simulink model "quadcopter_swarm_final_solution"  (R2023b)
settings: Solver=ode3  StartTime=0  StopTime=inf  FixedStep=0.005  RelTol=1e-3  EnableMultiTasking=on
values from neighbouring files (symbols this model uses):
  angle_outer_max = 60    [1nrx_dot.mat]    (also in 1nrxdrones_dot.mat; collision_avoidance_POS.mat; collision_avoidance_headonfix_POS.mat; collision_test.mat)
  F_e_g = [0 0 39.28]    [1nrx_dot.mat]    (also in 1nrxdrones_dot.mat; collision_avoidance_POS.mat; collision_avoidance_headonfix_POS.mat; collision_test.mat)
  g = 9.82    [1nrx_dot.mat]    (also in 1nrxdrones_dot.mat; collision_avoidance_POS.mat; collision_avoidance_headonfix_POS.mat; collision_test.mat)
  I_C = [0.5  0  0; 0  0.5  0; 0  0  1]    [1nrx_dot.mat]    (also in 1nrxdrones_dot.mat; collision_avoidance_POS.mat; collision_avoidance_headonfix_POS.mat; collision_test.mat)
  in_D = 20    [1nrx_dot.mat]    (also in 1nrxdrones_dot.mat; collision_avoidance_POS.mat; collision_avoidance_headonfix_POS.mat; collision_test.mat)
  in_I = 0    [1nrx_dot.mat]    (also in 1nrxdrones_dot.mat; collision_avoidance_POS.mat; collision_avoidance_headonfix_POS.mat; collision_test.mat)
  in_P = 20    [1nrx_dot.mat]    (also in 1nrxdrones_dot.mat; collision_avoidance_POS.mat; collision_avoidance_headonfix_POS.mat; collision_test.mat)
  in_thrust_D = 30    [1nrx_dot.mat]    (also in 1nrxdrones_dot.mat; collision_avoidance_POS.mat; collision_avoidance_headonfix_POS.mat; collision_test.mat)
  in_thrust_I = 0    [1nrx_dot.mat]    (also in 1nrxdrones_dot.mat; collision_avoidance_POS.mat; collision_avoidance_headonfix_POS.mat; collision_test.mat)
  in_thrust_P = 10    [1nrx_dot.mat]    (also in 1nrxdrones_dot.mat; collision_avoidance_POS.mat; collision_avoidance_headonfix_POS.mat; collision_test.mat)
  L = [4 -1 -1 -1 -1 0 -1 4 -1 -1 -1 0 ... (36 elements, 6x6)]    [1nrx_dot.mat]    (also in 1nrxdrones_dot.mat; collision_avoidance_POS.mat; collision_avoidance_headonfix_POS.mat; collision_test.mat)
  m = 4    [1nrx_dot.mat]    (also in 1nrxdrones_dot.mat; collision_avoidance_POS.mat; collision_avoidance_headonfix_POS.mat; collision_test.mat)
  M_RB = [4 0 0 0 0 0 0 4 0 0 0 0 ... (36 elements, 6x6)]    [1nrx_dot.mat]    (also in 1nrxdrones_dot.mat; collision_avoidance_POS.mat; collision_avoidance_headonfix_POS.mat; collision_test.mat)
  p_0 = [5  10; 5  -5; -8  5; 5  -13; 8  8; 0  0]    [1nrx_dot.mat]    (also in 1nrxdrones_dot.mat; collision_avoidance_POS.mat; collision_avoidance_headonfix_POS.mat; collision_test.mat)
  p_d = [1  0; 4  0; -2  0; 7  0; 9  0; 0  0]    [1nrx_dot.mat]    (also in 1nrxdrones_dot.mat; collision_avoidance_POS.mat; collision_avoidance_headonfix_POS.mat; collision_test.mat)
  R_c = 3    [1nrx_dot.mat]    (also in 1nrxdrones_dot.mat; collision_avoidance_POS.mat; collision_avoidance_headonfix_POS.mat; collision_test.mat)
  r_m = 2.2    [1nrx_dot.mat]    (also in 1nrxdrones_dot.mat; collision_avoidance_POS.mat; collision_avoidance_headonfix_POS.mat; collision_test.mat)
  thrust_max = 196.4    [1nrx_dot.mat]    (also in 1nrxdrones_dot.mat; collision_avoidance_POS.mat; collision_avoidance_headonfix_POS.mat; collision_test.mat)
  V = [1 2 3 4 5 6]    [1nrx_dot.mat]    (also in 1nrxdrones_dot.mat; collision_avoidance_POS.mat; collision_avoidance_headonfix_POS.mat; collision_test.mat)
  v_angle_in_max = 60    [1nrx_dot.mat]    (also in 1nrxdrones_dot.mat; collision_avoidance_POS.mat; collision_avoidance_headonfix_POS.mat; collision_test.mat)
  w = 0.6    [1nrx_dot.mat]    (also in 1nrxdrones_dot.mat; collision_avoidance_POS.mat; collision_avoidance_headonfix_POS.mat; collision_test.mat)
  w_1 = 6    [1nrx_dot.mat]    (also in 1nrxdrones_dot.mat; collision_avoidance_POS.mat; collision_avoidance_headonfix_POS.mat; collision_test.mat)
  w_2_with_h = 2.56430849099    [1nrx_dot.mat]    (also in 1nrxdrones_dot.mat; collision_avoidance_POS.mat; collision_avoidance_headonfix_POS.mat; collision_test.mat)
libraries: simulink_extras x37, slpidlib x30, sharedtransform x27, aerolibutil x25, dspsigops x24, dspindex x13, sharedutil x5, vrlib x2
(part 1 of 7)
settings Model: Creator=The MathWorks, Inc.  LastModifiedBy=Søren
settings SolverCC: AlgebraicLoopSolver=TrustRegion
settings DataIOCC: LimitDataPoints=on  SaveFormat=Array  SaveOutput=off  SignalLogging=off  DSMLogging=off  SaveTime=off  ReturnWorkspaceOutputs=off
settings OptimizationCC: BlockReduction=off  BufferReuse=off  LifeSpan=inf
settings DebuggingCC: AlgebraicLoopMsg=none  ParameterPrecisionLossMsg=none  AllowSymbolicDim=off  PregeneratedLibrarySubsystemCodeDiagnostic=none  SFUnexpectedBacktrackingDiag=warning  SFNoUnconditionalDefaultTransitionDiag=warning  SFExecutionAtInitializationDiag=none  ArithmeticOperatorsInVariantConditions=warning
settings HardwareCC: ProdBitPerPointer=32  ProdBitPerSizeT=32  ProdBitPerPtrDiffT=32  ProdLargestAtomicFloat=None  ProdIntDivRoundTo=Undefined  ProdEndianess=Unspecified  ProdWordSize=32  ProdHWDeviceType=32-bit Generic
settings ModelReferenceCC: EnableRefExpFcnMdlSchedulingChecks=on  PropagateSignalLabelsOutOfModel=off
settings SFSimCC: SimUseLocalCustomCode=off  CustomCodeUndefinedFunction=UseInterfaceOnly
settings RTWCC: RTWUseLocalCustomCode=off  DLArmComputeVersion=19.05
settings CodeAppCC: StateflowObjectComments=on
settings GRTTargetCC: TargetLangStandard=C89/C90 (ANSI)
settings ConfigComp: CovMetricSettings=dw  CovSaveCumulativeToWorkspaceVar=on  CovSaveSingleToWorkspaceVar=on  CovExternalEMLEnable=off  CovSFcnEnable=off

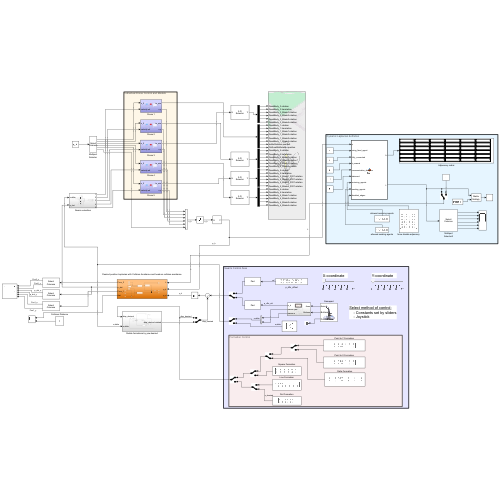
[thumbnail: Simulink's stored preview of the top-level diagram]
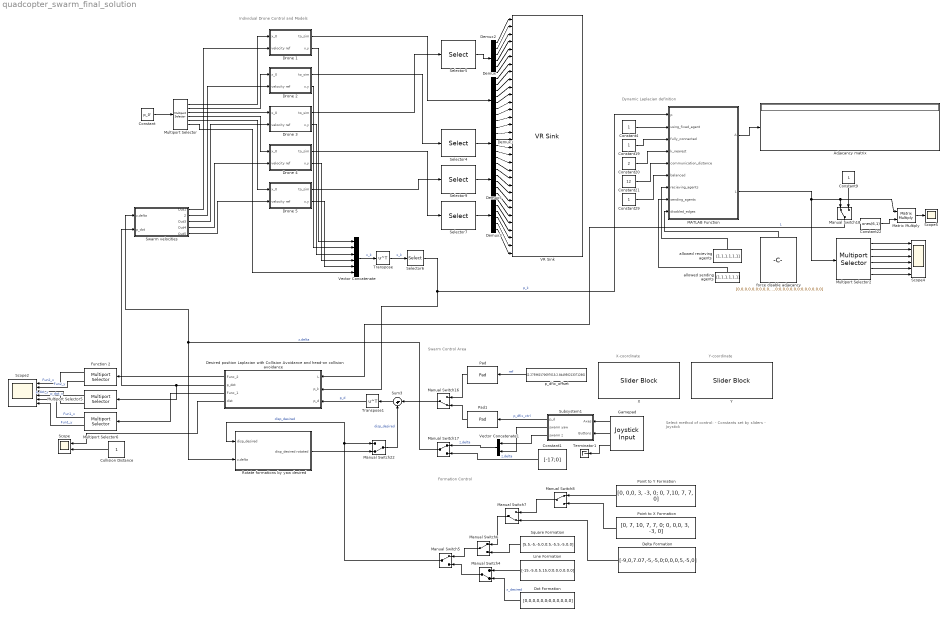
== system quadcopter_swarm_final_solution ==
  note: Individual Drone Control and Models
  note: Select method of control:
      | - Constants set by sliders
      | - Joystick
  note: Formation Control
  note: Swarm Control Area
  note: Dynamic Laplacian definition
  note: X-coordinate
  note: Y-coordinate
  Adjacancy matrix : Display
  Collision Distance : Constant
  Constant : Constant  Value=p_0'
  Constant1 : Constant  Value=[-17;0]  VectorParams1D=off
  Constant19 : Constant
  Constant20 : Constant  Value=2
  Constant21 : Constant  Value=12
  Constant22 : Constant  Value=ones(6,1)
  Constant29 : Constant
  Constant4 : Constant
  Constant9 : Constant  Value=L
  Delta Formation : Constant  Value=[-9,0,7.07,-5,-5,0;0,0,0,5,-5,0]
  Demux : Demux  Outputs=8
  Demux{1..3,5} (4 alike) : Demux  Outputs=6
  "Desired position Laplacian with Collision Avoidance and head-on collision avoidance " : Subsystem
  Dot Formation : Constant  Value=[0,0,0,0,0,0;0,0,0,0,0,0]
  Drone 1 : Subsystem
  Drone 2 : Subsystem
  Drone 3 : Subsystem
  Drone 4 : Subsystem
  Drone 5 : Subsystem
  Function 2 : dspindex/Multiport Selector  rowsOrCols=Columns  idxCellArray={ 1,2 }  idxErrMode=Clip Index
      settings: LibrarySourceBlock=|
      | dsphdlsupportsigmgmt/Multiport
      | Selector
  Gamepad : vrlib/Joystick Input  joyid=1  adjustports=on  forcefeed=off
  Line Formation : Constant  Value=[-15,-5,0,5,15,0;0,0,0,0,0,0]
  MATLAB Function : MATLAB Function  TreatAsAtomicUnit=on
  Manual Switch{4,7,16,22} (4 alike) : ManualSwitch  CurrentSetting=0
  Manual Switch{5..6,8,17..18} (5 alike) : ManualSwitch
  Matrix Multiply : Product  Multiplication=Matrix(*)
  Multiport Selector : dspindex/Multiport Selector  rowsOrCols=Columns  idxCellArray={1,2,3,4,5,6}  idxErrMode=Clip Index
      settings: LibrarySourceBlock=|
      | dsphdlsupportsigmgmt/Multiport
      | Selector
  Multiport Selector2 : dspindex/Multiport Selector  rowsOrCols=Columns  idxCellArray={ 1,2,3,4,5,6}  idxErrMode=Clip Index
      settings: LibrarySourceBlock=|
      | dsphdlsupportsigmgmt/Multiport
      | Selector
  Multiport Selector5 : dspindex/Multiport Selector  rowsOrCols=Columns  idxCellArray={ 1,2 }  idxErrMode=Clip Index
      settings: LibrarySourceBlock=|
      | dsphdlsupportsigmgmt/Multiport
      | Selector
  Multiport Selector6 : dspindex/Multiport Selector  rowsOrCols=Columns  idxCellArray={ 1,2 }  idxErrMode=Clip Index
      settings: LibrarySourceBlock=|
      | dsphdlsupportsigmgmt/Multiport
      | Selector
  Pad : dspsigops/Pad  padAlong=Rows  dimsToPad=1  valSrc=Specify via dialog  padVal=0  spec=Output size  padNumOutRowsSpecMethod=User-specified  numOutRows=2  padNumOutColsSpecMethod=User-specified  numOutCols=size(p_d,1)  isVarDimsMode=off  padBeginning=0  padEnd=0  outSizeMode=User-specified  outSize=1  padSigAt=Beginning  trunc_flag=None  roundingMode=Floor  overflowMode=off  truncOrWrapMode=Truncate  wrap_flag=None
  Pad1 : dspsigops/Pad  padAlong=Rows  dimsToPad=1  valSrc=Specify via dialog  padVal=0  spec=Output size  padNumOutRowsSpecMethod=User-specified  numOutRows=2  padNumOutColsSpecMethod=User-specified  numOutCols=size(p_d,1)  isVarDimsMode=off  padBeginning=0  padEnd=0  outSizeMode=User-specified  outSize=1  padSigAt=Beginning  trunc_flag=None  roundingMode=Floor  overflowMode=off  truncOrWrapMode=Truncate  wrap_flag=None
  Point to X Formation : Constant  Value=[0, 7, 10, 7, 7, 0; 0, 0,0, 3, -3, 0]
  Point to Y Formation : Constant  Value=[0, 0,0, 3, -3, 0; 0, 7,10, 7, 7, 0]
  Rotate formations by yaw desired : Subsystem
  Scope : Scope  NumInputPorts=2
  Scope2 : Scope  NumInputPorts=6
  Scope4 : Scope  NumInputPorts=6
  Scope5 : Scope
  Selector{4..5,7,9} (4 alike) : Selector  NumberOfDimensions=2  InputPortWidth=8  IndexOptions=Index vector (dialog),Select all  Indices=1:23,1  OutputSizes=1,1
  Selector6 : Selector  NumberOfDimensions=2  InputPortWidth=3  IndexOptions=Index vector (dialog),Select all  Indices=V,1  OutputSizes=1,1
  Square Formation : Constant  Value=[5,5,-5,-5,0,0;5,-5,5,-5,0,0]  VectorParams1D=off
  Subsystem1 : Subsystem
  Sum3 : Sum  Inputs=|-+
  Swarm velocities : Subsystem
  Terminator1 : Terminator
  Transpose : Math  Operator=transpose
  Transpose1 : Math  Operator=transpose
  VR Sink : vrlib/VR Sink  InstantiateOnLoad=on  SampleTime=12*0.005  ViewEnable=on  RemoteChange=off  RemoteView=off  FieldsWritten=QuadBody_3.rotation.4.1.1.double#QuadBody_3.translation.3.1.1.double#QuadBody_3_Blade1.rotation.4.1.1.double#QuadBody_3_Blade3.rotation.4.1.1.double#QuadBody_3_Blade2.rotation.4.1.1.double#QuadBody_3_Blade4.rotation.4.1.1.double#QuadBody_1.rotation.4.1.1.double#QuadBody_1.translation.3.1.1.double#QuadBody_1_Blade1.rotation.4.1.1.double#QuadBody_1_Blade3.rotation.4.1.1.double#QuadBody_1_Blade2.rotation.4.1.1.double#QuadBody_1_Blade4.rotation.4.1.1.double#IsoNoRotation.position.3.1.1.double#OnQuadNoRotation.position.3.1.1.double#QuadBody_2.rotation.4.1.1.double#QuadBody_2.translation.3.1.1.double#QuadBody_2_Blade1.rotation.4.1.1.double#QuadBody_2_Blade3.rotation.4.1.1.double#QuadBody_2_Blade2.rotation.4.1.1.double#QuadBody_2_Blade4.rotation.4.1.1.double#QuadBody_5.rotation.4.1.1.double#QuadBody_5.translation.3.1.1.double#QuadBody_5_Blade1_0001.rotation.4.1.1.double#QuadBody_5_Blade3_0001.rotation.4.1.1.double#QuadBody_5_Blade2_0001.rotation.4.1.1.double#QuadBody_5_Blade4_0001.rotation.4.1.1.double#QuadBody_4.rotation.4.1.1.double#QuadBody_4.translation.3.1.1.double#QuadBody_4_Blade1.rotation.4.1.1.double#QuadBody_4_Blade3.rotation.4.1.1.double#QuadBody_4_Blade2.rotation.4.1.1.double#QuadBody_4_Blade4.rotation.4.1.1.double  WorldFileName=Quadcopter_VR.wrl  AutoView=on  VideoDimensions=[]  AllowVariableSize=off  FigureProperties="{'Position', 'Name', 'Viewpoint', 'CameraBound', 'CameraDirection', 'CameraPosition', 'CameraUpVector', 'ZoomFactor', 'Antialiasing', 'Headlight', 'Lighting', 'NavPanel', 'Sound', 'StatusBar', 'Stereo3D', 'Stereo3DCameraOffset', 'Stereo3DHIT', 'ToolBar', 'Textures', 'Transparency', 'Triad', 'Wireframe', 'NavZones', 'NavMode', 'NavSpeed', 'CaptureFileFormat', 'CaptureFileName', 'Record2DCompressMethod', 'Record2DCompressQuality', 'Record2D', 'Record2DFileName', 'Record2DFPS'; [1.0000000000000000e+00   7.6000000000000000e+01   2.5600000000000000e+03   1.2650000000000000e+03], '', 'Chase Quad 5', 'on', [0.0000000000000000e+00   0.0000000000000000e+00  -1.0000000000000000e+00], [0.0000000000000000e+00   0.0000000000000000e+00   1.1000000000000000e+01], [0.0000000000000000e+00   1.0000000000000000e+00   0.0000000000000000e+00], [1.0000000000000000e+00], 'on', 'on', 'on', 'halfbar', 'on', 'on', 'off', [1.0000000149011612e-01], [0.0000000000000000e+00], 'on', 'on', 'on', 'none', 'off', 'off', 'fly', 'normal', 'tif', '%f_anim_%n.tif', 'auto', [7.5000000000000000e+01], 'off', '%f_anim_%n.avi', 'auto'}"
  Vector Concatenate : Concatenate  NumInputs=6  Mode=Multidimensional array  ConcatenateDimension=2
  Vector Concatenate1 : Concatenate  Mode=Multidimensional array
  X : SliderBlock  LabelPosition=Hide
  Y : SliderBlock  LabelPosition=Hide
  allowed recieving agents : Constant  Value=[1,1,1,1,1,1]
  allowed sending agents : Constant  Value=[1,1,1,1,1,1]
  force disable adjacancy : Constant  Value=[0,0,0,0,0,0;0,0,0,0,0,0;0,0,0,0,0,0;0,0,0,0,0,0;0,0,0,0,0,0;0,0,0,0,0,0]
  p_dfix_offset : Constant  Value=[2.275960170697013;2.844950213371266]  VectorParams1D=off
  wires:
  Selector5/1 -> Demux2/1
  Selector7/1 -> Demux3/1
  Selector4/1 -> Demux1/1
  Drone 1/2(x,y) -> Vector Concatenate/1
  Drone 2/2(x,y) -> Vector Concatenate/2
  Drone 3/2(x,y) -> Vector Concatenate/3
  Drone 4/2(x,y) -> Vector Concatenate/4
  Manual Switch17/1 -> Rotate formations by yaw desired/2(z,delta), Swarm velocities/1(z,delta)  "z,delta"
  Manual Switch22/1 -> Sum3/2  "disp_desired"
  Sum3/1 -> Transpose1/1
  Constant/1 -> Multiport Selector/1
  Vector Concatenate/1 -> Transpose/1  "x_k"
  Transpose/1 -> Selector6/1  "x_k"
  Multiport Selector/6 -> Vector Concatenate/6
  Manual Switch4/1 -> Manual Switch5/2
  Manual Switch6/1 -> Manual Switch5/1
  Dot Formation/1 -> Manual Switch4/2  "x_desired"
  Line Formation/1 -> Manual Switch4/1
  Square Formation/1 -> Manual Switch6/2
  Manual Switch7/1 -> Manual Switch6/1
  Delta Formation/1 -> Manual Switch7/2
  Point to Y Formation/1 -> Manual Switch8/1
  Point to X Formation/1 -> Manual Switch8/2
  Manual Switch8/1 -> Manual Switch7/1
  p_dfix_offset/1 -> Pad/1  "ref"
  Function 2/1 -> Scope2/1  "Fun2_x"
  Function 2/2 -> Scope2/2  "Fun2_y"
  Multiport Selector5/1 -> Scope2/3  "p_dot_x"
  Multiport Selector5/2 -> Scope2/4  "p_dot_y"
  Multiport Selector6/1 -> Scope2/5  "Fun1_x"
  Multiport Selector6/2 -> Scope2/6  "Fun1_y"
  Swarm velocities/1(Out1) -> Drone 1/2(velocity ref)
  Collision Distance/1 -> Scope/2
  Gamepad/1 -> Subsystem1/1(Axes)
  Gamepad/2 -> Subsystem1/2(Buttons)
  Manual Switch16/1 -> Sum3/1
  Pad/1 -> Manual Switch16/1
  Pad1/1 -> Manual Switch16/2
  Subsystem1/1(p_d) -> Pad1/1  "p_dfix_ctrl"
  Subsystem1/3(swarm z) -> Vector Concatenate1/1
  Drone 5/2(x,y) -> Vector Concatenate/5
  Demux2/1 -> VR Sink/1
  Demux2/2 -> VR Sink/2
  Demux2/3 -> VR Sink/3
  Demux2/4 -> VR Sink/4
  Demux2/5 -> VR Sink/5
  Demux2/6 -> VR Sink/6
  Demux/1 -> VR Sink/7
  Demux/2 -> VR Sink/8
  Demux/3 -> VR Sink/9
  Demux/4 -> VR Sink/10
  Demux/5 -> VR Sink/11
  Demux/6 -> VR Sink/12
  Demux/7 -> VR Sink/13
  Demux/8 -> VR Sink/14
  Demux1/1 -> VR Sink/15
  Demux1/2 -> VR Sink/16
  Demux1/3 -> VR Sink/17
  Demux1/4 -> VR Sink/18
  Demux1/5 -> VR Sink/19
  Demux1/6 -> VR Sink/20
  Demux3/1 -> VR Sink/27
  Demux3/2 -> VR Sink/28
  Demux3/3 -> VR Sink/29
  Demux3/4 -> VR Sink/30
  Demux3/5 -> VR Sink/31
  Demux3/6 -> VR Sink/32
  Demux5/2 -> VR Sink/22
  Demux5/5 -> VR Sink/25
  Demux5/1 -> VR Sink/21
  Demux5/6 -> VR Sink/26
  Demux5/3 -> VR Sink/23
  Demux5/4 -> VR Sink/24
  Selector9/1 -> Demux5/1
  Drone 1/1(to_sim) -> Demux/1
  Drone 2/1(to_sim) -> Selector4/1
  Drone 3/1(to_sim) -> Selector5/1
  Drone 4/1(to_sim) -> Selector7/1
  Drone 5/1(to_sim) -> Selector9/1
  Multiport Selector/1 -> Drone 1/1(x_0)
  Multiport Selector/2 -> Drone 2/1(x_0)
  Multiport Selector/3 -> Drone 3/1(x_0)
  Multiport Selector/4 -> Drone 4/1(x_0)
  Multiport Selector/5 -> Drone 5/1(x_0)
  Swarm velocities/2(2) -> Drone 2/2(velocity ref)
  Swarm velocities/3(Out3) -> Drone 3/2(velocity ref)
  Swarm velocities/4(Out4) -> Drone 4/2(velocity ref)
  Swarm velocities/5(Out5) -> Drone 5/2(velocity ref)
  Constant4/1 -> MATLAB Function/2(using_fixed_agent)
  Constant19/1 -> MATLAB Function/3(fully_connected)
  allowed recieving agents/1 -> MATLAB Function/7(recieving_agents)
  allowed sending agents/1 -> MATLAB Function/8(sending_agents)
  MATLAB Function/2(L) -> Multiport Selector2/1, Matrix Multiply/1, Manual Switch18/1
  Constant22/1 -> Matrix Multiply/2
  Matrix Multiply/1 -> Scope5/1
  Multiport Selector2/1 -> Scope4/1
  Multiport Selector2/2 -> Scope4/2
  Multiport Selector2/3 -> Scope4/3
  Multiport Selector2/4 -> Scope4/4
  Multiport Selector2/5 -> Scope4/5
  Multiport Selector2/6 -> Scope4/6
  Constant9/1 -> Manual Switch18/2
  Selector6/1 -> "Desired position Laplacian with Collision Avoidance and head-on collision avoidance "/2(p_k), MATLAB Function/1(p)  "p_k"
  Manual Switch5/1 -> Rotate formations by yaw desired/1(disp_desired), Manual Switch22/1  "disp_desired"
  MATLAB Function/1(A) -> Adjacancy matrix/1
  force disable adjacancy/1 -> MATLAB Function/9(disabled_edges)
  Constant20/1 -> MATLAB Function/4(k_nearest)
  Constant21/1 -> MATLAB Function/5(communication_distance)
  Constant29/1 -> MATLAB Function/6(balanced)
  Subsystem1/2(swarm yaw) -> Vector Concatenate1/2
  Constant1/1 -> Manual Switch17/2  "z,delta"
  Vector Concatenate1/1 -> Manual Switch17/1  "z,delta"
  "Desired position Laplacian with Collision Avoidance and head-on collision avoidance "/2(p_dot) -> Multiport Selector5/1, Swarm velocities/2(p_dot)
  Manual Switch18/1 -> "Desired position Laplacian with Collision Avoidance and head-on collision avoidance "/1(L)  "L"
  Transpose1/1 -> "Desired position Laplacian with Collision Avoidance and head-on collision avoidance "/3(p_d)  "p_d"
  "Desired position Laplacian with Collision Avoidance and head-on collision avoidance "/1(Func_2) -> Function 2/1
  "Desired position Laplacian with Collision Avoidance and head-on collision avoidance "/3(Func_1) -> Multiport Selector6/1
  "Desired position Laplacian with Collision Avoidance and head-on collision avoidance "/4(dist) -> Scope/1
  Rotate formations by yaw desired/1(disp_desired rotated) -> Manual Switch22/2
  Gamepad/3 -> Terminator1/1

== system quadcopter_swarm_final_solution/Desired position Laplacian with Collision Avoidance and head-on collision avoidance  ==
  L : Inport
  p_k : Inport  Port=2
  p_d : Inport  Port=3
  Collision Avoidance : MATLAB Function  TreatAsAtomicUnit=on
  Constant16 : Constant  Value=w_1
  Constant23 : Constant  Value=w_2_with_h
  Constant24 : Constant  Value=r_m
  Constant27 : Constant  Value=R_c
  Gain4 : Gain  Gain=w
  Head On Collision Solver : MATLAB Function  TreatAsAtomicUnit=on
  Sum : Sum  Inputs=--|+
  Sum10 : Sum  Inputs=+-|
  Swarm Velocities : MATLAB Function  TreatAsAtomicUnit=on
  Func_2 : Outport
  p_dot : Outport  Port=2
  Func_1 : Outport  Port=3
  dist : Outport  Port=4
  wires:
  Sum/1 -> Gain4/1  "p_dot"
  Head On Collision Solver/1(p_dot_h) -> Sum/1  "h"
  p_k/1 -> Sum10/1, Collision Avoidance/1(p)
  Constant27/1 -> Collision Avoidance/4(R_c)
  Collision Avoidance/1(p_dot_2) -> Sum/2, Func_2/1, Head On Collision Solver/1(fun2)  "Fun 2"
  Swarm Velocities/1(p_dot) -> Sum/3, Func_1/1  "Fun 1"
  Constant23/1 -> Collision Avoidance/2(w_2)
  Constant16/1 -> Swarm Velocities/2(w)
  Constant24/1 -> Collision Avoidance/3(r_m)
  Sum10/1 -> Swarm Velocities/1(delta_p)  "delta_p"
  Collision Avoidance/2(dist) -> dist/1
  Gain4/1 -> p_dot/1  "p_dot"
  L/1 -> Swarm Velocities/3(L)
  p_d/1 -> Sum10/2

== system quadcopter_swarm_final_solution/Drone 1 ==
  x_0 : Inport
  velocity ref : Inport  Port=2
  Constant5 : Constant  Value=[-45;0;0;0]  VectorParams1D=off
  Constant6 : Constant  Value=[20;20;20;20]  VectorParams1D=off
  Demux6 : Demux  Outputs=6
  Formatting : Subsystem
  Manual Switch : ManualSwitch  CurrentSetting=0
  Mux2 : Mux  Inputs=8
  PID controllers : Subsystem
  Pad : dspsigops/Pad  padAlong=Specified dimensions  dimsToPad=1  valSrc=Specify via dialog  padVal=0  spec=Output size  padNumOutRowsSpecMethod=User-specified  numOutRows=1  padNumOutColsSpecMethod=User-specified  numOutCols=6  isVarDimsMode=off  padBeginning=0  padEnd=0  outSizeMode=User-specified  outSize=6  padSigAt=Beginning  trunc_flag=None  roundingMode=Floor  overflowMode=off  truncOrWrapMode=Truncate  wrap_flag=None
  Quadcopter model Euler : Subsystem
  Radians to Degrees : simulink_extras/Transformations/Radians to Degrees
  Radians to Degrees1 : simulink_extras/Transformations/Radians to Degrees
  Radians to Degrees2 : simulink_extras/Transformations/Radians to Degrees
  Scope : Scope  NumInputPorts=3
  Scope1 : Scope  NumInputPorts=3
  Selector : Selector  InputPortWidth=6  IndexOptions=Index vector (dialog)  Indices=1:2  OutputSizes=1
  to_sim : Outport
  x,y : Outport  Port=2
  wires:
  Formatting/6(Position Blade 4) -> Mux2/6
  Demux6/1 -> Scope/1  "x"
  Demux6/6 -> Radians to Degrees2/1  "psi"
  Manual Switch/1 -> Quadcopter model Euler/1(tau_p)  "tau_p"
  Pad/1 -> Manual Switch/1  "tau_p_test"
  Demux6/5 -> Radians to Degrees1/1  "theta"
  Formatting/3(Position Blade1) -> Mux2/3
  Formatting/2(Out2) -> Mux2/2
  Demux6/4 -> Radians to Degrees/1  "phi"
  Demux6/3 -> Scope/3  "z"
  Constant6/1 -> Formatting/2(Propeller velocities)
  Constant5/1 -> Pad/1
  Demux6/2 -> Scope/2  "y"
  Formatting/7(Out7) -> Mux2/7
  Formatting/8(Out8) -> Mux2/8
  Formatting/5(Position Blade 3) -> Mux2/5
  Formatting/4(Position Blade 2) -> Mux2/4
  Formatting/1(Out1) -> Mux2/1
  PID controllers/1(tau_p) -> Manual Switch/2  "tau_p"
  Mux2/1 -> to_sim/1
  Quadcopter model Euler/1(eta) -> PID controllers/1(eta), Demux6/1, Selector/1, Formatting/1(Eta)
  x_0/1 -> Quadcopter model Euler/2(x_0)
  Quadcopter model Euler/2(eta_dot) -> PID controllers/2(eta_dot)
  velocity ref/1 -> PID controllers/3(velocity ref)
  Radians to Degrees/1 -> Scope1/1
  Radians to Degrees1/1 -> Scope1/2
  Radians to Degrees2/1 -> Scope1/3
  Selector/1 -> x,y/1

== system quadcopter_swarm_final_solution/Drone 2 ==
  x_0 : Inport
  velocity ref : Inport  Port=2
  Constant5 : Constant  Value=[-45;0;0;0]  VectorParams1D=off
  Constant6 : Constant  Value=[20;20;20;20]  VectorParams1D=off
  Demux6 : Demux  Outputs=6
  Formatting : Subsystem
  Manual Switch : ManualSwitch  CurrentSetting=0
  Mux2 : Mux  Inputs=8
  PID controllers : Subsystem
  Pad : dspsigops/Pad  padAlong=Specified dimensions  dimsToPad=1  valSrc=Specify via dialog  padVal=0  spec=Output size  padNumOutRowsSpecMethod=User-specified  numOutRows=1  padNumOutColsSpecMethod=User-specified  numOutCols=6  isVarDimsMode=off  padBeginning=0  padEnd=0  outSizeMode=User-specified  outSize=6  padSigAt=Beginning  trunc_flag=None  roundingMode=Floor  overflowMode=off  truncOrWrapMode=Truncate  wrap_flag=None
  Quadcopter model Euler : Subsystem
  Radians to Degrees : simulink_extras/Transformations/Radians to Degrees
  Radians to Degrees1 : simulink_extras/Transformations/Radians to Degrees
  Radians to Degrees2 : simulink_extras/Transformations/Radians to Degrees
  Scope : Scope  NumInputPorts=3
  Scope1 : Scope  NumInputPorts=3
  Selector : Selector  InputPortWidth=6  IndexOptions=Index vector (dialog)  Indices=1:2  OutputSizes=1
  to_sim : Outport
  x,y : Outport  Port=2
  wires:
  Formatting/6(Position Blade 4) -> Mux2/6
  Demux6/1 -> Scope/1  "x"
  Demux6/6 -> Radians to Degrees2/1  "psi"
  Manual Switch/1 -> Quadcopter model Euler/1(tau_p)  "tau_p"
  Pad/1 -> Manual Switch/1  "tau_p_test"
  Demux6/5 -> Radians to Degrees1/1  "theta"
  Formatting/3(Position Blade1) -> Mux2/3
  Formatting/2(Out2) -> Mux2/2
  Demux6/4 -> Radians to Degrees/1  "phi"
  Demux6/3 -> Scope/3  "z"
  Constant6/1 -> Formatting/2(Propeller velocities)
  Constant5/1 -> Pad/1
  Demux6/2 -> Scope/2  "y"
  Formatting/7(Out7) -> Mux2/7
  Formatting/8(Out8) -> Mux2/8
  Formatting/5(Position Blade 3) -> Mux2/5
  Formatting/4(Position Blade 2) -> Mux2/4
  Formatting/1(Out1) -> Mux2/1
  PID controllers/1(tau_p) -> Manual Switch/2  "tau_p"
  Mux2/1 -> to_sim/1
  Quadcopter model Euler/1(eta) -> PID controllers/1(eta), Demux6/1, Selector/1, Formatting/1(Eta)
  x_0/1 -> Quadcopter model Euler/2(x_0)
  Quadcopter model Euler/2(eta_dot) -> PID controllers/2(eta_dot)
  velocity ref/1 -> PID controllers/3(velocity ref)
  Radians to Degrees/1 -> Scope1/1
  Radians to Degrees1/1 -> Scope1/2
  Radians to Degrees2/1 -> Scope1/3
  Selector/1 -> x,y/1

== system quadcopter_swarm_final_solution/Drone 3 ==
  x_0 : Inport
  velocity ref : Inport  Port=2
  Constant5 : Constant  Value=[-45;0;0;0]  VectorParams1D=off
  Constant6 : Constant  Value=[20;20;20;20]  VectorParams1D=off
  Demux6 : Demux  Outputs=6
  Formatting : Subsystem
  Manual Switch : ManualSwitch  CurrentSetting=0
  Mux2 : Mux  Inputs=8
  PID controllers : Subsystem
  Pad : dspsigops/Pad  padAlong=Specified dimensions  dimsToPad=1  valSrc=Specify via dialog  padVal=0  spec=Output size  padNumOutRowsSpecMethod=User-specified  numOutRows=1  padNumOutColsSpecMethod=User-specified  numOutCols=6  isVarDimsMode=off  padBeginning=0  padEnd=0  outSizeMode=User-specified  outSize=6  padSigAt=Beginning  trunc_flag=None  roundingMode=Floor  overflowMode=off  truncOrWrapMode=Truncate  wrap_flag=None
  Quadcopter model Euler : Subsystem
  Radians to Degrees : simulink_extras/Transformations/Radians to Degrees
  Radians to Degrees1 : simulink_extras/Transformations/Radians to Degrees
  Radians to Degrees2 : simulink_extras/Transformations/Radians to Degrees
  Scope : Scope  NumInputPorts=3
  Scope1 : Scope  NumInputPorts=3
  Selector : Selector  InputPortWidth=6  IndexOptions=Index vector (dialog)  Indices=1:2  OutputSizes=1
  to_sim : Outport
  x,y : Outport  Port=2
  wires:
  Formatting/6(Position Blade 4) -> Mux2/6
  Demux6/1 -> Scope/1  "x"
  Demux6/6 -> Radians to Degrees2/1  "psi"
  Manual Switch/1 -> Quadcopter model Euler/1(tau_p)  "tau_p"
  Pad/1 -> Manual Switch/1  "tau_p_test"
  Demux6/5 -> Radians to Degrees1/1  "theta"
  Formatting/3(Position Blade1) -> Mux2/3
  Formatting/2(Out2) -> Mux2/2
  Demux6/4 -> Radians to Degrees/1  "phi"
  Demux6/3 -> Scope/3  "z"
  Constant6/1 -> Formatting/2(Propeller velocities)
  Constant5/1 -> Pad/1
  Demux6/2 -> Scope/2  "y"
  Formatting/7(Out7) -> Mux2/7
  Formatting/8(Out8) -> Mux2/8
  Formatting/5(Position Blade 3) -> Mux2/5
  Formatting/4(Position Blade 2) -> Mux2/4
  Formatting/1(Out1) -> Mux2/1
  PID controllers/1(tau_p) -> Manual Switch/2  "tau_p"
  Mux2/1 -> to_sim/1
  Quadcopter model Euler/1(eta) -> PID controllers/1(eta), Demux6/1, Selector/1, Formatting/1(Eta)
  x_0/1 -> Quadcopter model Euler/2(x_0)
  Quadcopter model Euler/2(eta_dot) -> PID controllers/2(eta_dot)
  velocity ref/1 -> PID controllers/3(velocity ref)
  Radians to Degrees/1 -> Scope1/1
  Radians to Degrees1/1 -> Scope1/2
  Radians to Degrees2/1 -> Scope1/3
  Selector/1 -> x,y/1

== system quadcopter_swarm_final_solution/Drone 4 ==
  x_0 : Inport
  velocity ref : Inport  Port=2
  Constant5 : Constant  Value=[-45;0;0;0]  VectorParams1D=off
  Constant6 : Constant  Value=[20;20;20;20]  VectorParams1D=off
  Demux6 : Demux  Outputs=6
  Formatting : Subsystem
  Manual Switch : ManualSwitch  CurrentSetting=0
  Mux2 : Mux  Inputs=8
  PID controllers : Subsystem
  Pad : dspsigops/Pad  padAlong=Specified dimensions  dimsToPad=1  valSrc=Specify via dialog  padVal=0  spec=Output size  padNumOutRowsSpecMethod=User-specified  numOutRows=1  padNumOutColsSpecMethod=User-specified  numOutCols=6  isVarDimsMode=off  padBeginning=0  padEnd=0  outSizeMode=User-specified  outSize=6  padSigAt=Beginning  trunc_flag=None  roundingMode=Floor  overflowMode=off  truncOrWrapMode=Truncate  wrap_flag=None
  Quadcopter model Euler : Subsystem
  Radians to Degrees : simulink_extras/Transformations/Radians to Degrees
  Radians to Degrees1 : simulink_extras/Transformations/Radians to Degrees
  Radians to Degrees2 : simulink_extras/Transformations/Radians to Degrees
  Scope : Scope  NumInputPorts=3
  Scope1 : Scope  NumInputPorts=3
  Selector : Selector  InputPortWidth=6  IndexOptions=Index vector (dialog)  Indices=1:2  OutputSizes=1
  to_sim : Outport
  x,y : Outport  Port=2
  wires:
  Formatting/6(Position Blade 4) -> Mux2/6
  Demux6/1 -> Scope/1  "x"
  Demux6/6 -> Radians to Degrees2/1  "psi"
  Manual Switch/1 -> Quadcopter model Euler/1(tau_p)  "tau_p"
  Pad/1 -> Manual Switch/1  "tau_p_test"
  Demux6/5 -> Radians to Degrees1/1  "theta"
  Formatting/3(Position Blade1) -> Mux2/3
  Formatting/2(Out2) -> Mux2/2
  Demux6/4 -> Radians to Degrees/1  "phi"
  Demux6/3 -> Scope/3  "z"
  Constant6/1 -> Formatting/2(Propeller velocities)
  Constant5/1 -> Pad/1
  Demux6/2 -> Scope/2  "y"
  Formatting/7(Out7) -> Mux2/7
  Formatting/8(Out8) -> Mux2/8
  Formatting/5(Position Blade 3) -> Mux2/5
  Formatting/4(Position Blade 2) -> Mux2/4
  Formatting/1(Out1) -> Mux2/1
  PID controllers/1(tau_p) -> Manual Switch/2  "tau_p"
  Mux2/1 -> to_sim/1
  Quadcopter model Euler/1(eta) -> PID controllers/1(eta), Demux6/1, Selector/1, Formatting/1(Eta)
  x_0/1 -> Quadcopter model Euler/2(x_0)
  Quadcopter model Euler/2(eta_dot) -> PID controllers/2(eta_dot)
  velocity ref/1 -> PID controllers/3(velocity ref)
  Radians to Degrees/1 -> Scope1/1
  Radians to Degrees1/1 -> Scope1/2
  Radians to Degrees2/1 -> Scope1/3
  Selector/1 -> x,y/1

== system quadcopter_swarm_final_solution/Drone 5 ==
  x_0 : Inport
  velocity ref : Inport  Port=2
  Constant5 : Constant  Value=[-45;0;0;0]  VectorParams1D=off
  Constant6 : Constant  Value=[20;20;20;20]  VectorParams1D=off
  Demux6 : Demux  Outputs=6
  Formatting : Subsystem
  Manual Switch : ManualSwitch  CurrentSetting=0
  Mux2 : Mux  Inputs=8
  PID controllers : Subsystem
  Pad : dspsigops/Pad  padAlong=Specified dimensions  dimsToPad=1  valSrc=Specify via dialog  padVal=0  spec=Output size  padNumOutRowsSpecMethod=User-specified  numOutRows=1  padNumOutColsSpecMethod=User-specified  numOutCols=6  isVarDimsMode=off  padBeginning=0  padEnd=0  outSizeMode=User-specified  outSize=6  padSigAt=Beginning  trunc_flag=None  roundingMode=Floor  overflowMode=off  truncOrWrapMode=Truncate  wrap_flag=None
  Quadcopter model Euler : Subsystem
  Radians to Degrees : simulink_extras/Transformations/Radians to Degrees
  Radians to Degrees1 : simulink_extras/Transformations/Radians to Degrees
  Radians to Degrees2 : simulink_extras/Transformations/Radians to Degrees
  Scope : Scope  NumInputPorts=3
  Scope1 : Scope  NumInputPorts=3
  Selector : Selector  InputPortWidth=6  IndexOptions=Index vector (dialog)  Indices=1:2  OutputSizes=1
  to_sim : Outport
  x,y : Outport  Port=2
  wires:
  Formatting/6(Position Blade 4) -> Mux2/6
  Demux6/1 -> Scope/1  "x"
  Demux6/6 -> Radians to Degrees2/1  "psi"
  Manual Switch/1 -> Quadcopter model Euler/1(tau_p)  "tau_p"
  Pad/1 -> Manual Switch/1  "tau_p_test"
  Demux6/5 -> Radians to Degrees1/1  "theta"
  Formatting/3(Position Blade1) -> Mux2/3
  Formatting/2(Out2) -> Mux2/2
  Demux6/4 -> Radians to Degrees/1  "phi"
  Demux6/3 -> Scope/3  "z"
  Constant6/1 -> Formatting/2(Propeller velocities)
  Constant5/1 -> Pad/1
  Demux6/2 -> Scope/2  "y"
  Formatting/7(Out7) -> Mux2/7
  Formatting/8(Out8) -> Mux2/8
  Formatting/5(Position Blade 3) -> Mux2/5
  Formatting/4(Position Blade 2) -> Mux2/4
  Formatting/1(Out1) -> Mux2/1
  PID controllers/1(tau_p) -> Manual Switch/2  "tau_p"
  Mux2/1 -> to_sim/1
  Quadcopter model Euler/1(eta) -> PID controllers/1(eta), Demux6/1, Selector/1, Formatting/1(Eta)
  x_0/1 -> Quadcopter model Euler/2(x_0)
  Quadcopter model Euler/2(eta_dot) -> PID controllers/2(eta_dot)
  velocity ref/1 -> PID controllers/3(velocity ref)
  Radians to Degrees/1 -> Scope1/1
  Radians to Degrees1/1 -> Scope1/2
  Radians to Degrees2/1 -> Scope1/3
  Selector/1 -> x,y/1

== system quadcopter_swarm_final_solution/Rotate formations by yaw desired ==
  disp_desired : Inport
  z,delta : Inport  Port=2
  Degrees to Radians : simulink_extras/Transformations/Degrees to Radians
  Ground : Ground
  Matrix Multiply3 : Product  Multiplication=Matrix(*)
  Mux2 : Mux  Inputs=3
  Pad2 : dspsigops/Pad  padAlong=Columns  dimsToPad=1  valSrc=Specify via dialog  padVal=0  spec=Output size  padNumOutRowsSpecMethod=User-specified  numOutRows=3  padNumOutColsSpecMethod=User-specified  numOutCols=3  isVarDimsMode=off  padBeginning=0  padEnd=0  outSizeMode=User-specified  outSize=1  padSigAt=End  trunc_flag=None  roundingMode=Floor  overflowMode=off  truncOrWrapMode=Truncate  wrap_flag=None
  Rotation Angles to Direction Cosine Matrix : sharedtransform/Rotation Angles to Direction Cosine Matrix  rotationOrder=ZYX  aMode=aMode
  Selector10 : Selector  InputPortWidth=2  IndexOptions=Index vector (dialog)  Indices=2  OutputSizes=1
  Selector11 : Selector  NumberOfDimensions=2  InputPortWidth=3  IndexOptions=Index vector (dialog),Select all  Indices=1:2,1:2  OutputSizes=1,1
  Transpose2 : Math  Operator=transpose
  disp_desired rotated : Outport
  wires:
  Matrix Multiply3/1 -> Selector11/1  "disp_desired rotated"
  Selector10/1 -> Degrees to Radians/1
  Transpose2/1 -> Matrix Multiply3/1
  Degrees to Radians/1 -> Mux2/1
  Rotation Angles to Direction Cosine Matrix/1 -> Transpose2/1
  disp_desired/1 -> Pad2/1
  Ground/1 -> Mux2/2, Mux2/3
  Pad2/1 -> Matrix Multiply3/2
  Mux2/1 -> Rotation Angles to Direction Cosine Matrix/1
  z,delta/1 -> Selector10/1
  Selector11/1 -> disp_desired rotated/1  "disp_desired rotated"

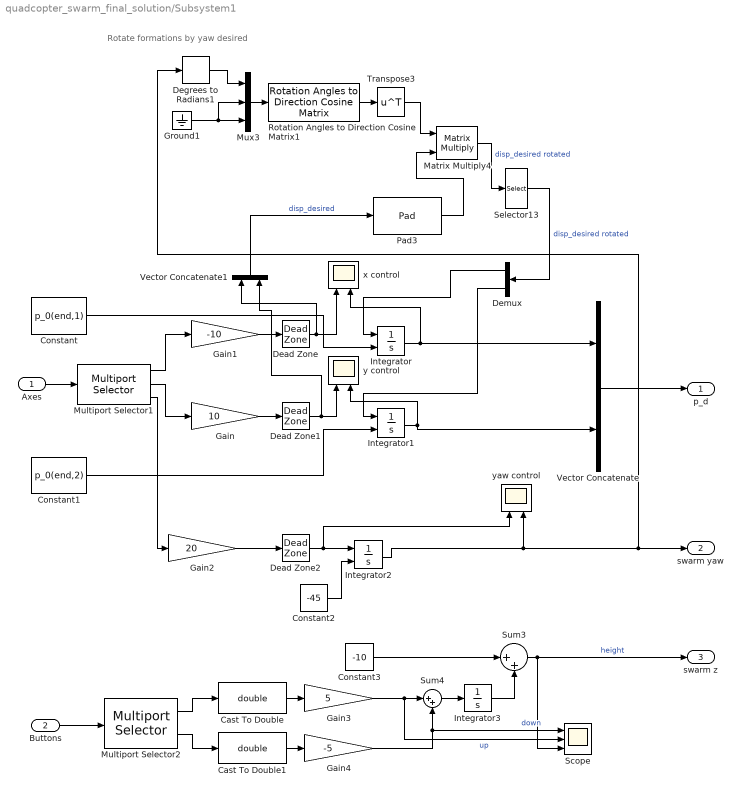
== system quadcopter_swarm_final_solution/Subsystem1 ==
  note: Rotate formations by yaw desired
  Axes : Inport
  Buttons : Inport  Port=2
  Cast To Double : DataTypeConversion  OutDataTypeStr=double  SaturateOnIntegerOverflow=off  RndMeth=Floor
  Cast To Double1 : DataTypeConversion  OutDataTypeStr=double  SaturateOnIntegerOverflow=off  RndMeth=Floor
  Constant : Constant  Value=p_0(end,1)
  Constant1 : Constant  Value=p_0(end,2)
  Constant2 : Constant  Value=-45
  Constant3 : Constant  Value=-10
  Dead Zone : DeadZone  LowerValue=-2  UpperValue=2
  Dead Zone1 : DeadZone  LowerValue=-2  UpperValue=2
  Dead Zone2 : DeadZone  LowerValue=-2  UpperValue=2
  Degrees to Radians1 : simulink_extras/Transformations/Degrees to Radians
  Demux : Demux  Outputs=2
  Gain : Gain  Gain=10
  Gain1 : Gain  Gain=-10
  Gain2 : Gain  Gain=20
  Gain3 : Gain  Gain=5
  Gain4 : Gain  Gain=-5
  Ground1 : Ground
  Integrator : Integrator  InitialConditionSource=external
  Integrator1 : Integrator  InitialConditionSource=external
  Integrator2 : Integrator  InitialConditionSource=external
  Integrator3 : Integrator
  Matrix Multiply4 : Product  Multiplication=Matrix(*)
  Multiport Selector1 : dspindex/Multiport Selector  rowsOrCols=Rows  idxCellArray={ 2, 1 , 3}  idxErrMode=Clip Index
      settings: LibrarySourceBlock=|
      | dsphdlsupportsigmgmt/Multiport
      | Selector
  Multiport Selector2 : dspindex/Multiport Selector  rowsOrCols=Rows  idxCellArray={ 5, 6}  idxErrMode=Clip Index
      settings: LibrarySourceBlock=|
      | dsphdlsupportsigmgmt/Multiport
      | Selector
  Mux3 : Mux  Inputs=3
  Pad3 : dspsigops/Pad  padAlong=Columns  dimsToPad=1  valSrc=Specify via dialog  padVal=0  spec=Output size  padNumOutRowsSpecMethod=User-specified  numOutRows=3  padNumOutColsSpecMethod=User-specified  numOutCols=3  isVarDimsMode=off  padBeginning=0  padEnd=0  outSizeMode=User-specified  outSize=1  padSigAt=End  trunc_flag=None  roundingMode=Floor  overflowMode=off  truncOrWrapMode=Truncate  wrap_flag=None
  Rotation Angles to Direction Cosine Matrix1 : sharedtransform/Rotation Angles to Direction Cosine Matrix  rotationOrder=ZYX  aMode=aMode
  Scope : Scope  NumInputPorts=3
  Selector13 : Selector  InputPortWidth=3  IndexOptions=Index vector (dialog)  Indices=1:2  OutputSizes=1
  Sum3 : Sum  Inputs=|++
  Sum4 : Sum  Inputs=|++
  Transpose3 : Math  Operator=transpose
  Vector Concatenate : Concatenate  Mode=Multidimensional array
  Vector Concatenate1 : Concatenate  Mode=Multidimensional array
  x control : Scope  NumInputPorts=2
  y control : Scope  NumInputPorts=2
  yaw control : Scope  NumInputPorts=2
  p_d : Outport
  swarm yaw : Outport  Port=2
  swarm z : Outport  Port=3
  wires:
  Vector Concatenate/1 -> p_d/1
  Buttons/1 -> Multiport Selector2/1
  Gain1/1 -> Dead Zone/1
  Dead Zone/1 -> x control/1, Vector Concatenate1/1
  Gain/1 -> Dead Zone1/1
  Dead Zone1/1 -> Vector Concatenate1/2, y control/1
  Integrator/1 -> Vector Concatenate/1, x control/2
  Integrator1/1 -> Vector Concatenate/2, y control/2
  Axes/1 -> Multiport Selector1/1
  Multiport Selector1/1 -> Gain1/1
  Multiport Selector1/2 -> Gain/1
  Gain2/1 -> Dead Zone2/1
  Multiport Selector1/3 -> Gain2/1
  Dead Zone2/1 -> Integrator2/1, yaw control/1
  Multiport Selector2/1 -> Cast To Double/1
  Multiport Selector2/2 -> Cast To Double1/1
  Gain3/1 -> Scope/2, Sum4/1  "up"
  Gain4/1 -> Scope/1, Sum4/2  "down"
  Sum3/1 -> Scope/3, swarm z/1  "height"
  Constant/1 -> Integrator/2
  Constant1/1 -> Integrator1/2
  Constant2/1 -> Integrator2/2
  Sum4/1 -> Integrator3/1
  Integrator3/1 -> Sum3/2
  Constant3/1 -> Sum3/1
  Cast To Double/1 -> Gain3/1
  Cast To Double1/1 -> Gain4/1
  Vector Concatenate1/1 -> Pad3/1  "disp_desired"
  Selector13/1 -> Demux/1  "disp_desired rotated"
  Rotation Angles to Direction Cosine Matrix1/1 -> Transpose3/1
  Matrix Multiply4/1 -> Selector13/1  "disp_desired rotated"
  Mux3/1 -> Rotation Angles to Direction Cosine Matrix1/1
  Degrees to Radians1/1 -> Mux3/1
  Pad3/1 -> Matrix Multiply4/2
  Ground1/1 -> Mux3/2, Mux3/3
  Integrator2/1 -> Degrees to Radians1/1, swarm yaw/1, yaw control/2
  Transpose3/1 -> Matrix Multiply4/1
  Demux/1 -> Integrator/1
  Demux/2 -> Integrator1/1

== system quadcopter_swarm_final_solution/Swarm velocities ==
  z,delta : Inport
  p_dot : Inport  Port=2
  Demux5 : Demux  Outputs=5
  Multiport Selector8 : dspindex/Multiport Selector  rowsOrCols=Columns  idxCellArray={1,2,3,4,5,6}  idxErrMode=Clip Index
      settings: LibrarySourceBlock=|
      | dsphdlsupportsigmgmt/Multiport
      | Selector
  Mux{1,12,14..16} (5 alike) : Mux  Inputs=2
  Mux13 : Mux  Inputs=5
  Terminator2 : Terminator
  Transpose3 : Math  Operator=transpose
  Out1 : Outport
  2 : Outport  Port=2
  Out3 : Outport  Port=3
  Out4 : Outport  Port=4
  Out5 : Outport  Port=5
  wires:
  Multiport Selector8/1 -> Mux12/1
  Mux12/1 -> Mux13/1
  z,delta/1 -> Mux12/2, Mux16/2, Mux1/2, Mux15/2, Mux14/2
  Mux14/1 -> Mux13/2
  Multiport Selector8/6 -> Terminator2/1
  Mux13/1 -> Demux5/1  "swarm velocities"
  Mux15/1 -> Mux13/3
  Transpose3/1 -> Multiport Selector8/1
  Multiport Selector8/2 -> Mux14/1
  Mux16/1 -> Mux13/4
  Multiport Selector8/3 -> Mux15/1
  Multiport Selector8/4 -> Mux16/1
  p_dot/1 -> Transpose3/1
  Demux5/1 -> Out1/1
  Demux5/2 -> 2/1
  Demux5/3 -> Out3/1
  Demux5/4 -> Out4/1
  Multiport Selector8/5 -> Mux1/1
  Mux1/1 -> Mux13/5
  Demux5/5 -> Out5/1

== system quadcopter_swarm_final_solution/Drone 1/Formatting ==
  Eta : Inport
  Propeller velocities : Inport  Port=2
  Axes to VR Axes : Subsystem
  Axes to VR Axes Camera Chase : Subsystem
  Axes to VR Axes Camera Iso : Subsystem
  Camera bias Chase : Bias  Bias=[-4 0 -.9558]'  SaturateOnIntegerOverflow=off
  Camera bias Iso : Bias  Bias=[0.9009 .99 -.6247]'  SaturateOnIntegerOverflow=off
  Demux : Demux  Outputs=6
  Euler to VR : Subsystem
  Mux1 : Mux  Inputs=3
  Mux3 : Mux  Inputs=3
  Rate Transition{,1..3} (4 alike) : RateTransition
  Subsystem : Subsystem
  Out1 : Outport
  Out2 : Outport  Port=2
  Position Blade1 : Outport  Port=3
  Position Blade 2 : Outport  Port=4
  Position Blade 3 : Outport  Port=5
  Position Blade 4 : Outport  Port=6
  Out7 : Outport  Port=7
  Out8 : Outport  Port=8
  wires:
  Rate Transition2/1 -> Out7/1
  Propeller velocities/1 -> Subsystem/1(Propeller velocities)
  Subsystem/3(Position Blade 3) -> Position Blade 3/1
  Subsystem/1(Position Blade1) -> Position Blade1/1
  Mux3/1 -> Euler to VR/1(Euler Angles)
  Camera bias Chase/1 -> Axes to VR Axes Camera Chase/1(Xe)
  Axes to VR Axes Camera Chase/1(Xe VR) -> Rate Transition3/1
  Subsystem/2(Position Blade 2) -> Position Blade 2/1
  Axes to VR Axes Camera Iso/1(Xe VR) -> Rate Transition2/1
  Euler to VR/1(Axis Angle) -> Rate Transition/1
  Axes to VR Axes/1(Xe VR) -> Rate Transition1/1
  Rate Transition1/1 -> Out2/1
  Camera bias Iso/1 -> Axes to VR Axes Camera Iso/1(Xe)
  Mux1/1 -> Camera bias Chase/1, Camera bias Iso/1, Axes to VR Axes/1(Xe)
  Rate Transition3/1 -> Out8/1
  Rate Transition/1 -> Out1/1
  Subsystem/4(Position Blade 4) -> Position Blade 4/1
  Demux/2 -> Mux1/2
  Demux/5 -> Mux3/2
  Demux/3 -> Mux1/3
  Eta/1 -> Demux/1
  Demux/1 -> Mux1/1
  Demux/4 -> Mux3/1
  Demux/6 -> Mux3/3

== system quadcopter_swarm_final_solution/Drone 1/PID controllers ==
  eta : Inport
  eta_dot : Inport  Port=2
  velocity ref : Inport  Port=3
  Inner-loop controllers : Subsystem
  Manual Switch : ManualSwitch
  Pad3 : dspsigops/Pad  padAlong=Rows  dimsToPad=1  valSrc=Specify via dialog  padVal=0  spec=Output size  padNumOutRowsSpecMethod=User-specified  numOutRows=1  padNumOutColsSpecMethod=User-specified  numOutCols=6  isVarDimsMode=off  padBeginning=0  padEnd=0  outSizeMode=User-specified  outSize=1  padSigAt=Beginning  trunc_flag=None  roundingMode=Floor  overflowMode=off  truncOrWrapMode=Truncate  wrap_flag=None
  Refs (alt. + Euler angles) : Constant  Value=[-10;0;0;0]  VectorParams1D=off
  Slider : SliderBlock  Commented=on  ScaleMin=-50  ScaleMax=50
  Slider1 : SliderBlock  Commented=on  ScaleMin=-50  ScaleMax=50
  Slider2 : SliderBlock  Commented=on  ScaleMin=-100
  outer-loop controllers output : Scope
  outer-loop velocity controller : Subsystem
  tau_p : Outport
  wires:
  outer-loop velocity controller/1(alt. + Euler angles) -> outer-loop controllers output/1, Manual Switch/1
  eta/1 -> Inner-loop controllers/2(eta), outer-loop velocity controller/3(eta)  "eta"
  Refs (alt. + Euler angles)/1 -> Manual Switch/2
  Manual Switch/1 -> Inner-loop controllers/1(refs)  "alt. + Euler angles"
  Pad3/1 -> tau_p/1
  Inner-loop controllers/1(Fz,mx,my,mz) -> Pad3/1
  eta_dot/1 -> outer-loop velocity controller/2(eta_dot)  "eta_dot"
  velocity ref/1 -> outer-loop velocity controller/1(velocity ref)

== system quadcopter_swarm_final_solution/Drone 1/Quadcopter model Euler ==
  tau_p : Inport
  x_0 : Inport  Port=2
  Gravity3 : Subsystem
  Quaternion-based kinematics : Subsystem
  Radians to Degrees3 : simulink_extras/Transformations/Radians to Degrees
  Scope1 : Scope  NumInputPorts=4
  Selector2 : Selector  InputPortWidth=6  IndexOptions=Index vector (dialog)  Indices=1:3  OutputSizes=1
  Sum : Sum  Inputs=|++
  rigid-body dynamics : Subsystem
  rotation scope : Scope
  eta : Outport
  eta_dot : Outport  Port=2
  wires:
  tau_p/1 -> Sum/1  "tau_p"
  Sum/1 -> rigid-body dynamics/1(tau), Scope1/1  "tau"
  rigid-body dynamics/1(nu_subsystem) -> Scope1/2, Quaternion-based kinematics/1(nu)  "nu"
  Radians to Degrees3/1 -> rotation scope/1  "rpy quaternion"
  Quaternion-based kinematics/2(eta_dot) -> eta_dot/1, Scope1/4  "eta_dot"
  Quaternion-based kinematics/1(eta) -> Selector2/1, eta/1, Scope1/3  "eta quaternion"
  Selector2/1 -> Radians to Degrees3/1
  x_0/1 -> Quaternion-based kinematics/2(x_0)
  Gravity3/1(tau_g) -> Sum/2
  Quaternion-based kinematics/3(R_b_e) -> Gravity3/1(R_b_e)

== system quadcopter_swarm_final_solution/Drone 2/Formatting ==
  Eta : Inport
  Propeller velocities : Inport  Port=2
  Axes to VR Axes : Subsystem
  Axes to VR Axes Camera Chase : Subsystem
  Axes to VR Axes Camera Iso : Subsystem
  Camera bias Chase : Bias  Bias=[-4 0 -.9558]'  SaturateOnIntegerOverflow=off
  Camera bias Iso : Bias  Bias=[0.9009 .99 -.6247]'  SaturateOnIntegerOverflow=off
  Demux : Demux  Outputs=6
  Euler to VR : Subsystem
  Mux1 : Mux  Inputs=3
  Mux3 : Mux  Inputs=3
  Rate Transition{,1..3} (4 alike) : RateTransition
  Subsystem : Subsystem
  Out1 : Outport
  Out2 : Outport  Port=2
  Position Blade1 : Outport  Port=3
  Position Blade 2 : Outport  Port=4
  Position Blade 3 : Outport  Port=5
  Position Blade 4 : Outport  Port=6
  Out7 : Outport  Port=7
  Out8 : Outport  Port=8
  wires:
  Rate Transition2/1 -> Out7/1
  Propeller velocities/1 -> Subsystem/1(Propeller velocities)
  Subsystem/3(Position Blade 3) -> Position Blade 3/1
  Subsystem/1(Position Blade1) -> Position Blade1/1
  Mux3/1 -> Euler to VR/1(Euler Angles)
  Camera bias Chase/1 -> Axes to VR Axes Camera Chase/1(Xe)
  Axes to VR Axes Camera Chase/1(Xe VR) -> Rate Transition3/1
  Subsystem/2(Position Blade 2) -> Position Blade 2/1
  Axes to VR Axes Camera Iso/1(Xe VR) -> Rate Transition2/1
  Euler to VR/1(Axis Angle) -> Rate Transition/1
  Axes to VR Axes/1(Xe VR) -> Rate Transition1/1
  Rate Transition1/1 -> Out2/1
  Camera bias Iso/1 -> Axes to VR Axes Camera Iso/1(Xe)
  Mux1/1 -> Camera bias Chase/1, Camera bias Iso/1, Axes to VR Axes/1(Xe)
  Rate Transition3/1 -> Out8/1
  Rate Transition/1 -> Out1/1
  Subsystem/4(Position Blade 4) -> Position Blade 4/1
  Demux/2 -> Mux1/2
  Demux/5 -> Mux3/2
  Demux/3 -> Mux1/3
  Eta/1 -> Demux/1
  Demux/1 -> Mux1/1
  Demux/4 -> Mux3/1
  Demux/6 -> Mux3/3

== system quadcopter_swarm_final_solution/Drone 2/PID controllers ==
  eta : Inport
  eta_dot : Inport  Port=2
  velocity ref : Inport  Port=3
  Inner-loop controllers : Subsystem
  Manual Switch : ManualSwitch
  Pad3 : dspsigops/Pad  padAlong=Rows  dimsToPad=1  valSrc=Specify via dialog  padVal=0  spec=Output size  padNumOutRowsSpecMethod=User-specified  numOutRows=1  padNumOutColsSpecMethod=User-specified  numOutCols=6  isVarDimsMode=off  padBeginning=0  padEnd=0  outSizeMode=User-specified  outSize=1  padSigAt=Beginning  trunc_flag=None  roundingMode=Floor  overflowMode=off  truncOrWrapMode=Truncate  wrap_flag=None
  Refs (alt. + Euler angles) : Constant  Value=[-10;0;0;0]  VectorParams1D=off
  Slider : SliderBlock  Commented=on  ScaleMin=-50  ScaleMax=50
  Slider1 : SliderBlock  Commented=on  ScaleMin=-50  ScaleMax=50
  Slider2 : SliderBlock  Commented=on  ScaleMin=-100
  outer-loop controllers output : Scope
  outer-loop velocity controller : Subsystem
  tau_p : Outport
  wires:
  outer-loop velocity controller/1(alt. + Euler angles) -> outer-loop controllers output/1, Manual Switch/1
  eta/1 -> Inner-loop controllers/2(eta), outer-loop velocity controller/3(eta)  "eta"
  Refs (alt. + Euler angles)/1 -> Manual Switch/2
  Manual Switch/1 -> Inner-loop controllers/1(refs)  "alt. + Euler angles"
  Pad3/1 -> tau_p/1
  Inner-loop controllers/1(Fz,mx,my,mz) -> Pad3/1
  eta_dot/1 -> outer-loop velocity controller/2(eta_dot)  "eta_dot"
  velocity ref/1 -> outer-loop velocity controller/1(velocity ref)

== system quadcopter_swarm_final_solution/Drone 2/Quadcopter model Euler ==
  tau_p : Inport
  x_0 : Inport  Port=2
  Gravity3 : Subsystem
  Quaternion-based kinematics : Subsystem
  Radians to Degrees3 : simulink_extras/Transformations/Radians to Degrees
  Scope1 : Scope  NumInputPorts=4
  Selector2 : Selector  InputPortWidth=6  IndexOptions=Index vector (dialog)  Indices=1:3  OutputSizes=1
  Sum : Sum  Inputs=|++
  rigid-body dynamics : Subsystem
  rotation scope : Scope
  eta : Outport
  eta_dot : Outport  Port=2
  wires:
  tau_p/1 -> Sum/1  "tau_p"
  Sum/1 -> rigid-body dynamics/1(tau), Scope1/1  "tau"
  rigid-body dynamics/1(nu_subsystem) -> Scope1/2, Quaternion-based kinematics/1(nu)  "nu"
  Radians to Degrees3/1 -> rotation scope/1  "rpy quaternion"
  Quaternion-based kinematics/2(eta_dot) -> eta_dot/1, Scope1/4  "eta_dot"
  Quaternion-based kinematics/1(eta) -> Selector2/1, eta/1, Scope1/3  "eta quaternion"
  Selector2/1 -> Radians to Degrees3/1
  x_0/1 -> Quaternion-based kinematics/2(x_0)
  Gravity3/1(tau_g) -> Sum/2
  Quaternion-based kinematics/3(R_b_e) -> Gravity3/1(R_b_e)

== system quadcopter_swarm_final_solution/Drone 3/Formatting ==
  Eta : Inport
  Propeller velocities : Inport  Port=2
  Axes to VR Axes : Subsystem
  Axes to VR Axes Camera Chase : Subsystem
  Axes to VR Axes Camera Iso : Subsystem
  Camera bias Chase : Bias  Bias=[-4 0 -.9558]'  SaturateOnIntegerOverflow=off
  Camera bias Iso : Bias  Bias=[0.9009 .99 -.6247]'  SaturateOnIntegerOverflow=off
  Demux : Demux  Outputs=6
  Euler to VR : Subsystem
  Mux1 : Mux  Inputs=3
  Mux3 : Mux  Inputs=3
  Rate Transition{,1..3} (4 alike) : RateTransition
  Subsystem : Subsystem
  Out1 : Outport
  Out2 : Outport  Port=2
  Position Blade1 : Outport  Port=3
  Position Blade 2 : Outport  Port=4
  Position Blade 3 : Outport  Port=5
  Position Blade 4 : Outport  Port=6
  Out7 : Outport  Port=7
  Out8 : Outport  Port=8
  wires:
  Rate Transition2/1 -> Out7/1
  Propeller velocities/1 -> Subsystem/1(Propeller velocities)
  Subsystem/3(Position Blade 3) -> Position Blade 3/1
  Subsystem/1(Position Blade1) -> Position Blade1/1
  Mux3/1 -> Euler to VR/1(Euler Angles)
  Camera bias Chase/1 -> Axes to VR Axes Camera Chase/1(Xe)
  Axes to VR Axes Camera Chase/1(Xe VR) -> Rate Transition3/1
  Subsystem/2(Position Blade 2) -> Position Blade 2/1
  Axes to VR Axes Camera Iso/1(Xe VR) -> Rate Transition2/1
  Euler to VR/1(Axis Angle) -> Rate Transition/1
  Axes to VR Axes/1(Xe VR) -> Rate Transition1/1
  Rate Transition1/1 -> Out2/1
  Camera bias Iso/1 -> Axes to VR Axes Camera Iso/1(Xe)
  Mux1/1 -> Camera bias Chase/1, Camera bias Iso/1, Axes to VR Axes/1(Xe)
  Rate Transition3/1 -> Out8/1
  Rate Transition/1 -> Out1/1
  Subsystem/4(Position Blade 4) -> Position Blade 4/1
  Demux/2 -> Mux1/2
  Demux/5 -> Mux3/2
  Demux/3 -> Mux1/3
  Eta/1 -> Demux/1
  Demux/1 -> Mux1/1
  Demux/4 -> Mux3/1
  Demux/6 -> Mux3/3
